simulink model "model2"  (R2022a)
settings: Solver=FixedStepAuto  StartTime=0.0  StopTime=10.0  FixedStep=1  RelTol=1e-3
values from neighbouring files (symbols this model uses):
  path = [0 0 0 0 0 0 0 0 0 0 0 0 ... (18 elements, 9x2)]    [aufgabe2.mat]    (also in createPath.m = pathTemp)
  testMap = [0  0  0; 0  1  0; 0  0  0]    [aufgabe2.mat]
settings Model: Creator=JadKHaddad  LastModifiedBy=JadKHaddad

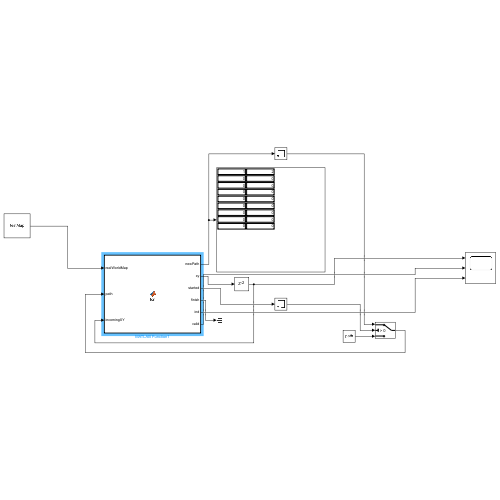
[thumbnail: Simulink's stored preview of the top-level diagram]
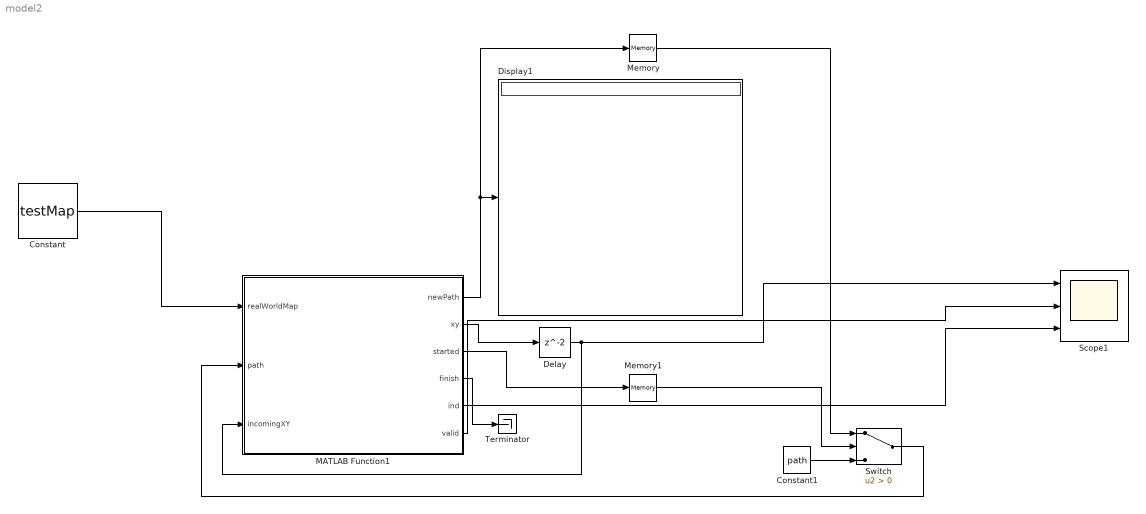
== system model2 ==
  Constant : Constant  Value=testMap  VectorParams1D=off
  Constant1 : Constant  Value=path  VectorParams1D=off
  Delay : Delay
  Display1 : Display
  MATLAB Function1 : MATLAB Function  TreatAsAtomicUnit=on
  Memory : Memory
  Memory1 : Memory
  Scope1 : Scope  NumInputPorts=3
  Switch : Switch  Criteria=u2 > Threshold  SaturateOnIntegerOverflow=off  InputSameDT=off
  Terminator : Terminator
  wires:
  MATLAB Function1/3(started) -> Memory1/1
  Constant1/1 -> Switch/3
  MATLAB Function1/2(xy) -> Delay/1
  MATLAB Function1/4(finish) -> Terminator/1
  Switch/1 -> MATLAB Function1/2(path)
  Memory/1 -> Switch/1
  Memory1/1 -> Switch/2
  MATLAB Function1/1(newPath) -> Memory/1, Display1/1
  Delay/1 -> MATLAB Function1/3(incomingXY), Scope1/1
  MATLAB Function1/5(ind) -> Scope1/3
  Constant/1 -> MATLAB Function1/1(realWorldMap)
  MATLAB Function1/6(valid) -> Scope1/2

== matlab function model2/MATLAB Function1 ==
  data: realWorldMap input; path input; newPath output; xy output; started output; finish output; incomingXY input; ind output; valid output
function [newPath, xy, started, finish, ind, valid] = fcn(realWorldMap, path, incomingXY)
    persistent index
    persistent limit


    if isempty(index)
        index = 1;
    end

    
    if isempty(limit)
        limit = 2;
    end
    started = 1;
    finish = 0;
    
    xy = path(1,:);
    valid = 0;
    if index > length(path)
        finish = 1;
    else
        if index < limit
            valid = 1;
            index = index + 1;
            x = incomingXY(1, 1) + 1;
            y = incomingXY(1, 1) + 1;
            if realWorldMap(x,y) == 0
                if x + 1 <= length(realWorldMap) && realWorldMap(x + 1, y) == 0 && containsFunc(path, x+1, y) == 0
                    newRow = [x+1 y];
                    path(limit-1,:) = newRow;
                    limit = limit + 1;
                end
                
                if y + 1 <= length(realWorldMap) && realWorldMap(x, y + 1) == 0 && containsFunc(path, x, y + 1) == 0
                    newRow = [x y+1];
                    path(limit-1,:) = newRow;
                    limit = limit + 1;
                end
                
                if x - 1 >= 1 && realWorldMap(x - 1, y) == 0 && containsFunc(path, x - 1, y) == 0
                    newRow = [x-1 y];
                    path(limit-1,:) = newRow;
                    limit = limit + 1;
                end
                
                if y - 1 >= 1 && realWorldMap(x, y-1) == 0 && containsFunc(path, x, y-1) == 0
                    newRow = [x y-1];
                    path(limit-1,:) = newRow;
                    limit = limit + 1;
                end
           
            end
        end

        
        
    end
    
    newPath = path;
    ind = index;
